simulink model "Flyback_Master"  (R2019b)
settings: Solver=VariableStepAuto  StartTime=0.0  StopTime=10.0  RelTol=1e-3
libraries: powerlib x8
settings Model: Creator=Chitra Manis Raja  LastModifiedBy=Chitra Manis Raja

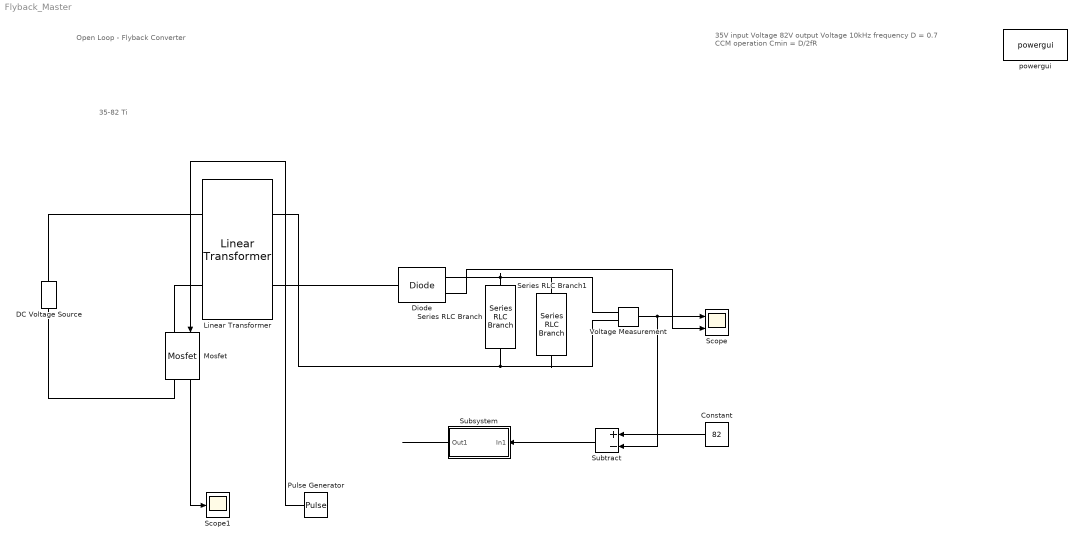
== system Flyback_Master ==
  note: 35-82 Ti
  note: Open Loop - Flyback Converter
  note: 35V input Voltage
      | 82V output Voltage
      | 10kHz frequency
      | D = 0.7
      | CCM operation
      | Cmin = D/2fR
  Constant : Constant  Value=82
  DC Voltage Source : powerlib/Electrical Sources/DC Voltage Source  Amplitude=35  Measurements=None
      settings: SourceProductName=Simscape Electrical
  Diode : powerlib/Power Electronics/Diode  Ron=0.001  Lon=0  Vf=0.8  IC=0  UseSnubber=0  Rs=500  Cs=250e-9  Measurements=on
      settings: SourceProductName=Simscape Electrical
  Linear Transformer : powerlib/Elements/Linear Transformer  UNITS=SI  NominalPower=[ 70 10e3 ]  winding1=[35 0 30e-6]  winding2=[35 0 0]  ThreeWindings=off  winding3=[3.15e+05 3.969e+07 6316.9]  RmLm=[1e4 1000e-6]  Measurements=None  DataType=on
      settings: SourceProductName=Simscape Electrical
  Mosfet : powerlib/Power Electronics/Mosfet  Ron=0.1  Lon=0  Rd=0.01  Vfd=0  IC=0  Rs=1e5  Cs=inf  Measurements=on
      settings: SourceProductName=Simscape Electrical
  Pulse Generator : DiscretePulseGenerator  PulseType=Time based  Period=1/10e3  PulseWidth=70
  Scope : Scope  NumInputPorts=2
  Scope1 : Scope
  Series RLC Branch : powerlib/Elements/Series RLC Branch  LConnTagsString=__new0  RConnTagsString=__new0  BranchType=C  Resistance=1  Inductance=1e-3  SetiL0=off  InitialCurrent=0  Capacitance=300e-6  Setx0=off  InitialVoltage=0  Measurements=None
      settings: SourceProductName=Simscape Electrical
  Series RLC Branch1 : powerlib/Elements/Series RLC Branch  LConnTagsString=__new0  RConnTagsString=__new0  BranchType=R  Resistance=100  Inductance=1e-3  SetiL0=off  InitialCurrent=0  Capacitance=1e-6  Setx0=off  InitialVoltage=0  Measurements=None
      settings: SourceProductName=Simscape Electrical
  Subsystem : Subsystem
  Subtract : Sum  Inputs=+-
  Voltage Measurement : powerlib/Measurements/Voltage Measurement  PhasorSimulation=off  OutputType=Complex  PSBequivalent=0
      settings: SourceProductName=Simscape Electrical
  powergui : powerlib/powergui  Priority=1  SimulationMode=Continuous  SampleTime=50e-6  frequency=60  Iterations=50  frequencyindice=0  Pbase=100e6  ErrMax=1e-4  UnitsV=kV  UnitsW=MW  buscounter=0  FunctionMessages=off  echomessages=off  EnableUseOfTLC=off  CurrentSourceSwitches=off  DisableSnubberDevices=off  DisableRonSwitches=off  DisableVfSwitches=off  DisplayEquations=off  AutomaticDiscreteSolvers=off  SolverType=Tustin/Backward Euler (TBE)  Interpol=off  ExternalGateDelay=off  methode=off  Ts=100  x0status=blocks  SPID=on  SwTol=0  HookPort=off  NonlinearTolerance=1e-4  nMaxIteration=100  ContinueOnMaxIteration=off  RestoreLinks=warning  ResistiveCurrentMeasurement=off  Frange=[0:2:500]  Ylog=off  Xlog=on  ShowGrid=off  save=off  variable=ZData  structure=0  ZoomFFT=off  StartTime=0.0  cycles=1  DisplayStyle=1  fundamental=60  FreqAxis=off  MaxFrequency=1000  frequencyindicesteady=1  RmsSteady=1  display=off
      settings: SourceProductName=Simscape Electrical
  wires:
  Pulse Generator/1 -> Mosfet/1
  Mosfet/1 -> Scope1/1
  Voltage Measurement/1 -> Subtract/2, Scope/1
  Diode/1 -> Scope/2
  Constant/1 -> Subtract/1
  Subtract/1 -> Subsystem/1(In1)
  Subsystem/1(Out1) -> ?
  connections:
  Linear Transformer/LConn1 -- DC Voltage Source/RConn1
  Series RLC Branch/RConn1 -- Voltage Measurement/LConn2 -- Series RLC Branch1/RConn1 -- Linear Transformer/RConn1
  Diode/LConn1 -- Linear Transformer/RConn2
  Linear Transformer/LConn2 -- Mosfet/LConn1
  Mosfet/RConn1 -- DC Voltage Source/LConn1
  Series RLC Branch/LConn1 -- Voltage Measurement/LConn1 -- Series RLC Branch1/LConn1 -- Diode/RConn1

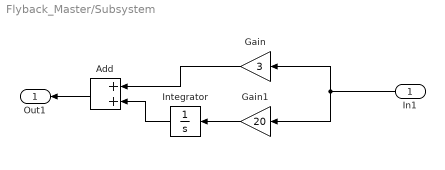
== system Flyback_Master/Subsystem ==
  In1 : Inport
  Add : Sum
  Gain : Gain  Gain=3
  Gain1 : Gain  Gain=20
  Integrator : Integrator
  Out1 : Outport
  wires:
  Gain1/1 -> Integrator/1
  Integrator/1 -> Add/2
  Gain/1 -> Add/1
  In1/1 -> Gain1/1, Gain/1
  Add/1 -> Out1/1
